simulink model "longitudinalControl2"  (R2020b)
settings: Solver=VariableStepAuto  StartTime=0.0  StopTime=tsim  RelTol=1e-3
values from neighbouring files (symbols this model uses):
  Af = -1/tau    (= -1000)    [main.m]
  Bf = 1/tau    (= 1000)    [main.m]
  Cf = 1    [main.m]
  Cr = 0.01    [main.m]
  Cv = 0.32    [Comfort-orientedCruise_Control.m]    (also in main.m)
  Da = 1.3    [main.m]
  delay = 0    [main.m]
  FMax = 4000    [Comfort-orientedCruise_Control.m]    (also in main.m = 5000)
  g = 9.81    [Comfort-orientedCruise_Control.m]    (also in main.m)
  K1 = (Y1*inv(Q))    [LQRLMI_cvx.m]
  K2 = (Y2*inv(Q))    [LQRLMI_cvx.m]
  K3 = (Y3*inv(Q))    [LQRLMI_cvx.m]
  K4 = (Y4*inv(Q))    [LQRLMI_cvx.m]
  rho1Max = 1/1400    (= 0.000714285714286)    [main.m]
  rho1Min = 1/1680    (= 0.000595238095238)    [main.m]
  rho2Max = 35    [main.m]
  rho2Min = 0    [main.m]
  S = 2.4    [main.m]
  tauAct = 0    [main.m]
  tsim = 120    [main.m]
  v0 = 11    [main.m]
  windAve = 12/3.6    (= 3.33333333333)    [main.m]
undefined symbols (not defined in the file or in its folder): initialSpeeds, vRefComputer
libraries: simulink x5
settings Model: Creator=DELL  LastModifiedBy=DELL

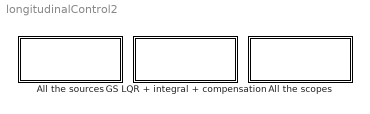
== system longitudinalControl2 ==
  All the scopes : Subsystem
  All the sources : Subsystem
  GS LQR + integral + compensation : Subsystem

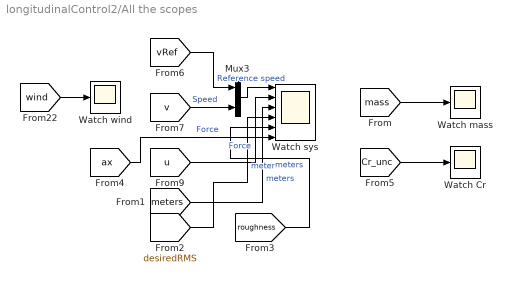
== system longitudinalControl2/All the scopes ==
  Mux3 : Mux  Inputs=2
  Watch Cr : Scope
  Watch mass : Scope
  Watch sys : Scope  NumInputPorts=6
  Watch wind : Scope
  wires:
  [vRef] -> Mux3/1  "Reference speed"
  Mux3/1 -> Watch sys/1
  [v] -> Mux3/2  "Speed"
  [u] -> Watch sys/2  "Force"
  [wind] -> Watch wind/1
  [meters] -> Watch sys/3  "meters"
  [desiredRMS] -> Watch sys/4  "meters"
  [roughness] -> Watch sys/5  "meters"
  [ax] -> Watch sys/6  "Force"
  [mass] -> Watch mass/1
  [Cr_unc] -> Watch Cr/1

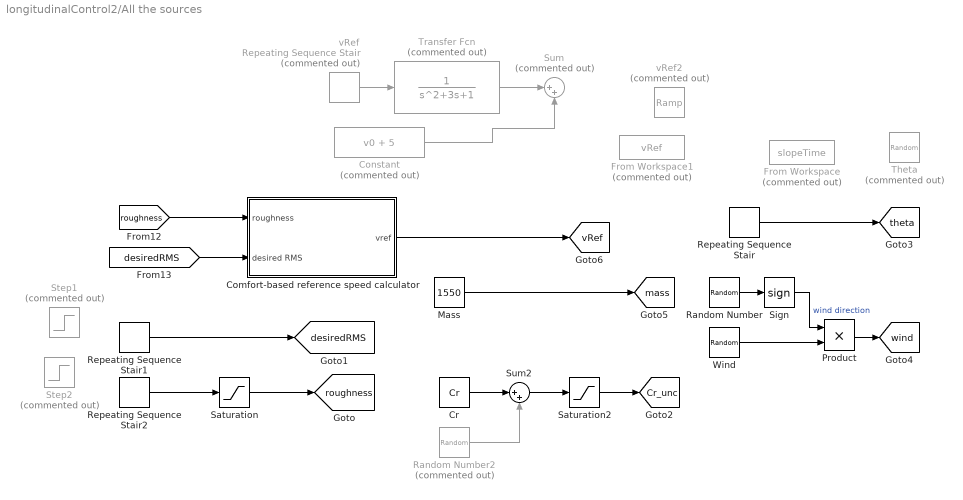
== system longitudinalControl2/All the sources ==
  Comfort-based reference speed calculator : Subsystem
  Constant : Constant  Commented=on  Value=v0 + 5
  Cr : Constant  Value=Cr
  From Workspace : FromWorkspace  Commented=on  VariableName=slopeTime
  From Workspace1 : FromWorkspace  Commented=on  VariableName=vRef
  Mass : Constant  Value=1550
  Product : Product
  Random Number : RandomNumber  Variance=0.1  SampleTime=1
  Random Number2 : RandomNumber  Commented=on  Variance=0.0000005  SampleTime=5
  Repeating Sequence Stair : simulink/Sources/Repeating Sequence Stair  OutValues=(pi/1800)*[0 3 6 3 0 -3 -6 -3].'  tsamp=0.5  OutMin=[]  OutMax=[]  OutDataTypeStr=double  OutputDataTypeScalingMode=double  OutDataType=fixdt(0,8)  ConRadixGroup=Best Precision: Vector-wise  OutScaling=2^-12
  Repeating Sequence Stair1 : simulink/Sources/Repeating Sequence Stair  OutValues=[0.3 0.2 0.2 0.4 0.3] + [0.2 0.4 0.4 0.3 0.2]*0  tsamp=tsim/5  OutMin=[]  OutMax=[]  OutDataTypeStr=double  OutputDataTypeScalingMode=double  OutDataType=fixdt(0,8)  ConRadixGroup=Best Precision: Vector-wise  OutScaling=2^-12
  Repeating Sequence Stair2 : simulink/Sources/Repeating Sequence Stair  OutValues=1e-6*[30 30 3 3 30] + 1e-6*[3 3 30 30 3]*0  tsamp=tsim/5  OutMin=[]  OutMax=[]  OutDataTypeStr=double  OutputDataTypeScalingMode=double  OutDataType=fixdt(0,8)  ConRadixGroup=Best Precision: Vector-wise  OutScaling=2^-12
  Saturation : Saturate  UpperLimit=1617e-6  LowerLimit=0
  Saturation2 : Saturate  UpperLimit=0.012  LowerLimit=0.008
  Sign : Signum
  Step1 : Step  Commented=on  Time=tsim/3  Before=0.2  After=0.3  SampleTime=0
  Step2 : Step  Commented=on  Time=2*tsim/3  Before=5e-6*0 + 30e-6  After=20e-6*0 + 3e-6  SampleTime=0
  Sum : Sum  Commented=on  Inputs=|++
  Sum2 : Sum  Inputs=|++
  Theta : RandomNumber  Commented=on  Variance=0.1  SampleTime=0.1
  Transfer Fcn : TransferFcn  Commented=on  Denominator=[1 3 1]
  Wind : RandomNumber  Mean=windAve  Variance=10  SampleTime=1
  vRef : simulink/Sources/Repeating Sequence Stair  Commented=on  OutValues=[-10 0].'  tsamp=40  OutMin=[]  OutMax=[]  OutDataTypeStr=double  OutputDataTypeScalingMode=double  OutDataType=fixdt(0,8)  ConRadixGroup=Best Precision: Vector-wise  OutScaling=2^-12
  vRef2 : simulink/Sources/Ramp  Commented=on  slope=0.5  start=0  InitialOutput=0
  tag scope: Cr_unc=global, desiredRMS=global, mass=global, roughness=global, theta=global, vRef=global, wind=global
  wires:
  Random Number/1 -> Sign/1
  Wind/1 -> Product/2
  Sign/1 -> Product/1  "wind direction"
  Product/1 -> [wind]
  Repeating Sequence Stair/1 -> [theta]
  Transfer Fcn/1 -> Sum/1
  vRef/1 -> Transfer Fcn/1
  Constant/1 -> Sum/2
  [desiredRMS] -> Comfort-based reference speed calculator/2(desired RMS)
  [roughness] -> Comfort-based reference speed calculator/1(roughness)
  Saturation/1 -> [roughness]
  Repeating Sequence Stair1/1 -> [desiredRMS]
  Repeating Sequence Stair2/1 -> Saturation/1
  Comfort-based reference speed calculator/1(vref) -> [vRef]
  Mass/1 -> [mass]
  Cr/1 -> Sum2/1
  Sum2/1 -> Saturation2/1
  Saturation2/1 -> [Cr_unc]
  Random Number2/1 -> Sum2/2

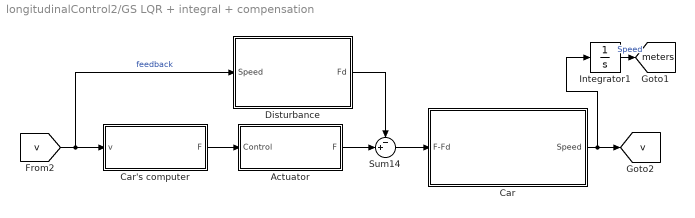
== system longitudinalControl2/GS LQR + integral + compensation ==
  Actuator : Subsystem
  Car : Subsystem
  Car's computer : Subsystem
  Disturbance : Subsystem
  Integrator1 : Integrator
  Sum14 : Sum  Inputs=-+|
  tag scope: meters=global, v=global
  wires:
  Disturbance/1(Fd) -> Sum14/1
  [v] -> Disturbance/1(Speed), Car's computer/1(v)  "feedback"
  Actuator/1(F) -> Sum14/2
  Sum14/1 -> Car/1("F-Fd ")
  Car's computer/1(F) -> Actuator/1(Control)
  Integrator1/1 -> [meters]  "Speed"
  Car/1(Speed) -> Integrator1/1, [v]

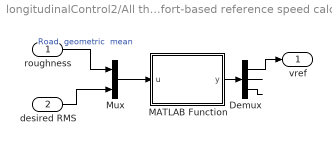
== system longitudinalControl2/All the sources/Comfort-based reference speed calculator ==
  roughness : Inport
  desired RMS : Inport  Port=2
  Demux : Demux  Outputs=3
  MATLAB Function : MATLAB Function  TreatAsAtomicUnit=on
  Mux : Mux  Inputs=2
  vref : Outport  VectorParamsAs1DForOutWhenUnconnected=off
  wires:
  Mux/1 -> MATLAB Function/1(u)
  MATLAB Function/1(y) -> Demux/1
  Demux/2 -> ?
  Demux/3 -> ?
  Demux/1 -> vref/1
  roughness/1 -> Mux/1  "Road  geometric  mean"
  desired RMS/1 -> Mux/2

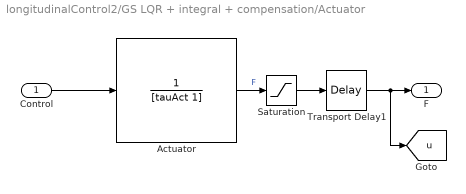
== system longitudinalControl2/GS LQR + integral + compensation/Actuator ==
  Control : Inport
  Actuator : TransferFcn  Denominator=[tauAct 1]
  Saturation : Saturate  UpperLimit=FMax  LowerLimit=-FMax
  Transport Delay1 : TransportDelay  DelayTime=delay
  F : Outport  VectorParamsAs1DForOutWhenUnconnected=off
  tag scope: u=global
  wires:
  Control/1 -> Actuator/1
  Saturation/1 -> Transport Delay1/1
  Actuator/1 -> Saturation/1  "F"
  Transport Delay1/1 -> [u], F/1

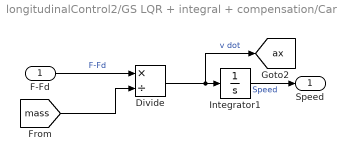
== system longitudinalControl2/GS LQR + integral + compensation/Car ==
  "F-Fd " : Inport
  Divide : Product  Inputs=*/
  Integrator1 : Integrator  InitialCondition=v0
  Speed : Outport  VectorParamsAs1DForOutWhenUnconnected=off
  tag scope: ax=global
  wires:
  Divide/1 -> [ax], Integrator1/1  "v dot"
  "F-Fd "/1 -> Divide/1  "F-Fd"
  [mass] -> Divide/2
  Integrator1/1 -> Speed/1  "Speed"

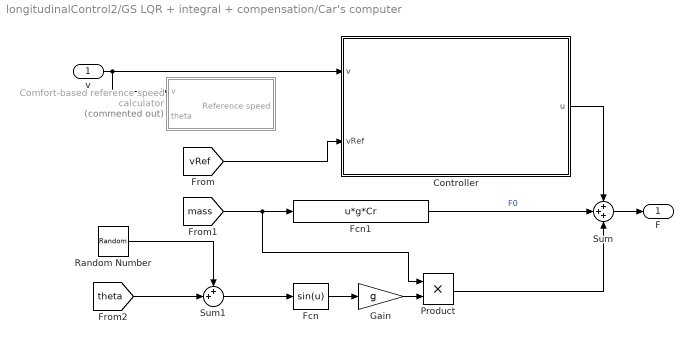
== system longitudinalControl2/GS LQR + integral + compensation/Car's computer ==
  v : Inport
  Comfort-based reference speed calculator : Subsystem  Commented=on
  Controller : Subsystem
  Fcn : Fcn  Expr=sin(u)
  Fcn1 : Fcn  Expr=u*g*Cr
  Gain : Gain  Gain=g
  Product : Product
  Random Number : RandomNumber  Variance=0.00001  SampleTime=0.1
  Sum : Sum  Inputs=+++
  Sum1 : Sum  Inputs=++|
  F : Outport  VectorParamsAs1DForOutWhenUnconnected=off
  wires:
  v/1 -> Comfort-based reference speed calculator/1(v), Controller/1(v)
  [vRef] -> Controller/2(vRef)
  Controller/1(u) -> Sum/1
  Sum/1 -> F/1
  [mass] -> Product/1, Fcn1/1
  Fcn/1 -> Gain/1
  Fcn1/1 -> Sum/2  "F0"
  Gain/1 -> Product/2
  [theta] -> Sum1/2
  Sum1/1 -> Fcn/1
  Random Number/1 -> Sum1/1
  Product/1 -> Sum/3

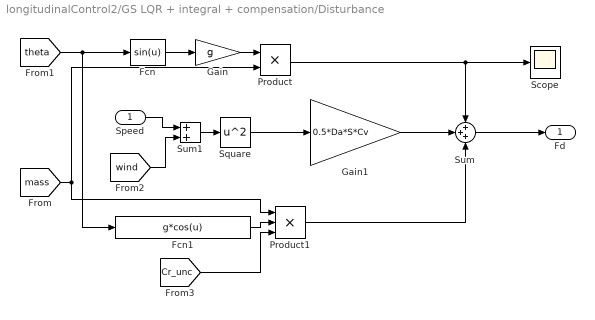
== system longitudinalControl2/GS LQR + integral + compensation/Disturbance ==
  Speed : Inport
  Fcn : Fcn  Expr=sin(u)
  Fcn1 : Fcn  Expr=g*cos(u)
  Gain : Gain  Gain=g
  Gain1 : Gain  Gain=0.5*Da*S*Cv
  Product : Product
  Product1 : Product  Inputs=3
  Scope : Scope
  Square : Math  Operator=square  SignedPower=on  SaturateOnIntegerOverflow=on
  Sum : Sum  Inputs=+++
  Sum1 : Sum
  Fd : Outport  VectorParamsAs1DForOutWhenUnconnected=off
  wires:
  [wind] -> Sum1/2
  Product1/1 -> Sum/3
  Fcn1/1 -> Product1/2
  [mass] -> Product/2, Product1/1
  Gain/1 -> Product/1
  Product/1 -> Sum/1, Scope/1
  Speed/1 -> Sum1/1
  Sum1/1 -> Square/1
  Fcn/1 -> Gain/1
  Sum/1 -> Fd/1
  Gain1/1 -> Sum/2
  Square/1 -> Gain1/1
  [theta] -> Fcn/1, Fcn1/1
  [Cr_unc] -> Product1/3

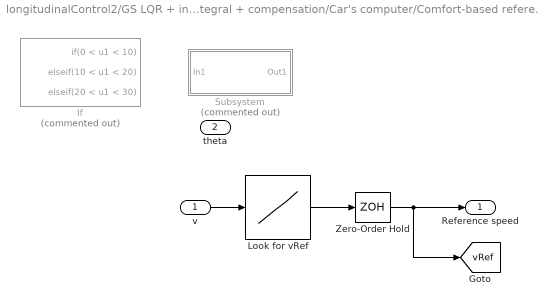
== system longitudinalControl2/GS LQR + integral + compensation/Car's computer/Comfort-based reference speed calculator ==
  v : Inport
  theta : Inport  Port=2
  If : If  Commented=on  IfExpression=0 < u1 < 10  ElseIfExpressions=10 < u1 < 20, 20 < u1 < 30  ShowElse=off
  Look for vRef : Lookup_n-D  NumberOfTableDimensions=1  BreakpointsForDimension1=initialSpeeds  BreakpointsForDimension2=initialSpeeds  Table=vRefComputer(:, 1)  InternalRulePriority=Speed  RndMeth=Simplest  InputSameDT=on
  Subsystem : Subsystem  Commented=on
  Zero-Order Hold : ZeroOrderHold  SampleTime=10
  Reference speed : Outport  VectorParamsAs1DForOutWhenUnconnected=off
  tag scope: vRef=global
  wires:
  v/1 -> Look for vRef/1
  Look for vRef/1 -> Zero-Order Hold/1
  Zero-Order Hold/1 -> [vRef], Reference speed/1

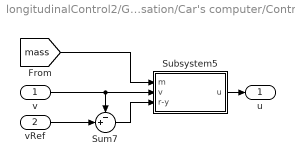
== system longitudinalControl2/GS LQR + integral + compensation/Car's computer/Controller ==
  v : Inport
  vRef : Inport  Port=2
  Subsystem5 : Subsystem
  Sum7 : Sum  Inputs=-+|
  u : Outport  VectorParamsAs1DForOutWhenUnconnected=off
  wires:
  vRef/1 -> Sum7/2
  v/1 -> Subsystem5/2(v), Sum7/1
  Subsystem5/1(u) -> u/1
  [mass] -> Subsystem5/1(m)
  Sum7/1 -> Subsystem5/3(r-y)

== system longitudinalControl2/GS LQR + integral + compensation/Car's computer/Comfort-based reference speed calculator/Subsystem ==
  In1 : Inport
  Out1 : Outport  VectorParamsAs1DForOutWhenUnconnected=off

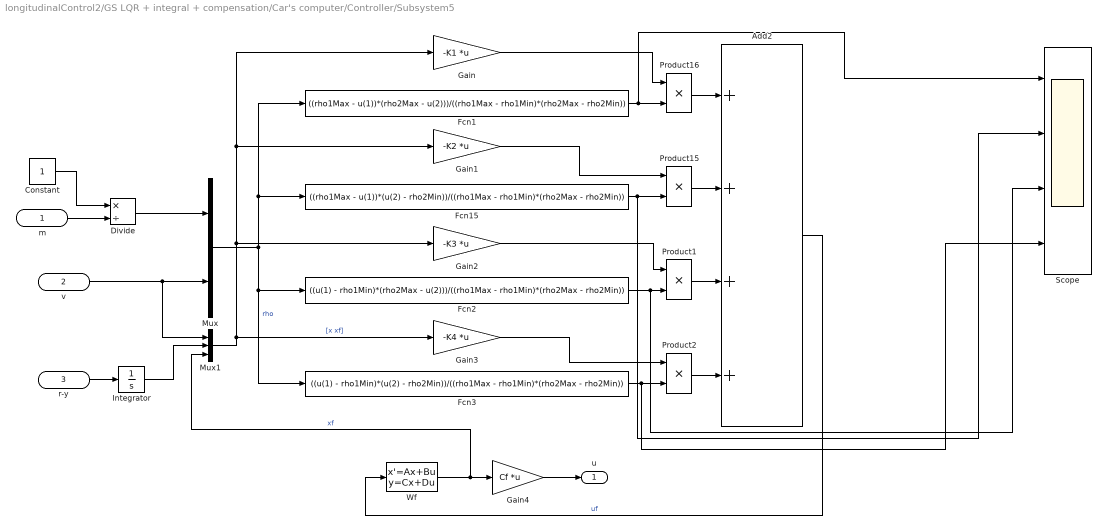
== system longitudinalControl2/GS LQR + integral + compensation/Car's computer/Controller/Subsystem5 ==
  m : Inport
  v : Inport  Port=2
  r-y : Inport  Port=3
  Add2 : Sum  Inputs=++++
  Constant : Constant
  Divide : Product  Inputs=*/
  Fcn1 : Fcn  Expr=((rho1Max - u(1))*(rho2Max - u(2)))/((rho1Max - rho1Min)*(rho2Max - rho2Min))
  Fcn15 : Fcn  Expr=((rho1Max - u(1))*(u(2) - rho2Min))/((rho1Max - rho1Min)*(rho2Max - rho2Min))
  Fcn2 : Fcn  Expr=((u(1) - rho1Min)*(rho2Max - u(2)))/((rho1Max - rho1Min)*(rho2Max - rho2Min))
  Fcn3 : Fcn  Expr=((u(1) - rho1Min)*(u(2) - rho2Min))/((rho1Max - rho1Min)*(rho2Max - rho2Min))
  Gain : Gain  Gain=-K1  Multiplication=Matrix(K*u) (u vector)
  Gain1 : Gain  Gain=-K2  Multiplication=Matrix(K*u) (u vector)
  Gain2 : Gain  Gain=-K3  Multiplication=Matrix(K*u) (u vector)
  Gain3 : Gain  Gain=-K4  Multiplication=Matrix(K*u) (u vector)
  Gain4 : Gain  Gain=Cf  Multiplication=Matrix(K*u) (u vector)
  Integrator : Integrator
  Mux : Mux  Inputs=2
  Mux1 : Mux  Inputs=3
  Product{1..2,15..16} (4 alike) : Product  RndMeth=Zero
  Scope : Scope  NumInputPorts=4
  Wf : StateSpace  A=Af  B=Bf  D=0  InitialCondition=0
  u : Outport  VectorParamsAs1DForOutWhenUnconnected=off
  wires:
  Gain/1 -> Product16/1
  Gain1/1 -> Product15/1
  Product15/1 -> Add2/2
  Product16/1 -> Add2/1
  Fcn15/1 -> Scope/2, Product15/2
  Fcn1/1 -> Scope/1, Product16/2
  Gain2/1 -> Product1/1
  Product1/1 -> Add2/3
  Fcn2/1 -> Scope/3, Product1/2
  Gain3/1 -> Product2/1
  Product2/1 -> Add2/4
  Fcn3/1 -> Scope/4, Product2/2
  v/1 -> Mux1/1, Mux/2
  Mux/1 -> Fcn1/1, Fcn15/1, Fcn3/1, Fcn2/1  "rho"
  Divide/1 -> Mux/1
  m/1 -> Divide/2
  Constant/1 -> Divide/1
  Integrator/1 -> Mux1/2
  r-y/1 -> Integrator/1
  Mux1/1 -> Gain3/1, Gain/1, Gain1/1, Gain2/1  "[x xf]"
  Wf/1 -> Mux1/3, Gain4/1  "xf"
  Gain4/1 -> u/1
  Add2/1 -> Wf/1  "uf"

== matlab function longitudinalControl2/All the sources/Comfort-based reference speed calculator/MATLAB Function ==
  data: u input; y output
function y = fcn(u)
poli_road_A =[-2.810588227248419e+05,6.169326456562061e+05,-5.532877354090116e+05,2.592697706189919e+05,-6.700633721138796e+04,9.126098470124590e+03,-4.908206795592492e+02,17.034337618461410];
poli_road_B=[-2.918464207163787e+03,1.256660289518003e+04,-2.213392570093140e+04,2.042007729169009e+04,-1.043888402402951e+04,2.839027450728016e+03,-3.194031408439325e+02,20.363551425734784];
poli_road_C=[-20.580699008933195,1.768188289251797e+02,-6.209471832216163e+02,1.140851851658809e+03,-1.158899742214876e+03,6.230583939060465e+02,-1.343821697265132e+02,17.843722322086556];
poli_road_D=[-0.189767159734969,3.220641909579672,-22.334773208111000,81.060950477925270,-1.629224058712685e+02,1.740926522486322e+02,-76.471563472280050,19.565680049932546];
rho=u(1);
comf=u(2);
vref=0;
if (0 <= rho) & (rho <= 6.3e-6)
   vref=polyval(poli_road_A,comf);
elseif (12.3e-6 < rho) & (rho <= 25.3e-6)
    vref=polyval(poli_road_B,comf);
elseif (25.3e-6 < rho) & (rho <= 101.1e-6)
    vref=polyval(poli_road_C,comf);
elseif (101.1e-6 < rho) & (rho <= 404.3e-6)
    vref=polyval(poli_road_D,comf);
end
y=[vref;rho;comf];
